simulink model "mil_top"  (R2025b)
settings: Solver=FixedStepDiscrete  StartTime=0.0  StopTime=mil_t_final_s  FixedStep=0.01  RelTol=1e-3
settings Model: Creator=O.Agaphonov  LastModifiedBy=O.Agaphonov

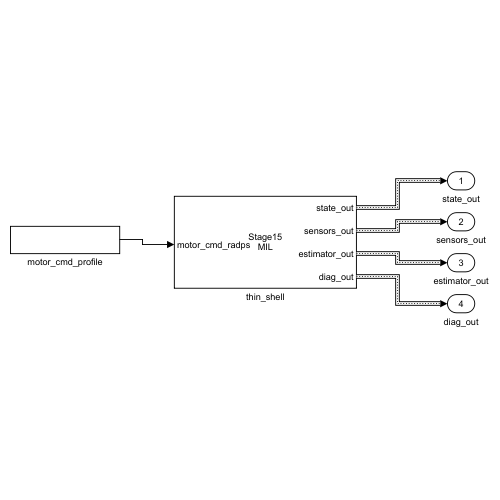
[thumbnail: Simulink's stored preview of the top-level diagram]
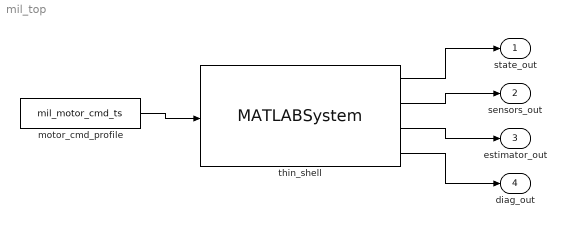
== system mil_top ==
  motor_cmd_profile : FromWorkspace  VariableName=mil_motor_cmd_ts
  thin_shell : MATLABSystem  System=uav.sl.Stage15MILSystem  dt_s=mil_dt_s  state0=mil_state0  params=mil_params  SimulateUsing=Interpreted execution
      mask Type: uav.sl.Stage15MILSystem
  state_out : Outport
  sensors_out : Outport  Port=2
  estimator_out : Outport  Port=3
  diag_out : Outport  Port=4
  wires:
  motor_cmd_profile/1 -> thin_shell/1
  thin_shell/1 -> state_out/1
  thin_shell/2 -> sensors_out/1
  thin_shell/3 -> estimator_out/1
  thin_shell/4 -> diag_out/1
